simulink library "wopc_lib"  (R2024b)
settings: Solver=VariableStepAuto  StartTime=0.0  StopTime=10.0  RelTol=1e-3
undefined symbols (not defined in the file or in its folder): lambda_1, lambda_3, omega, vessel
libraries: $bdroot x13, mssSimulink x2
settings Model: Creator=lenna  LastModifiedBy=lenna

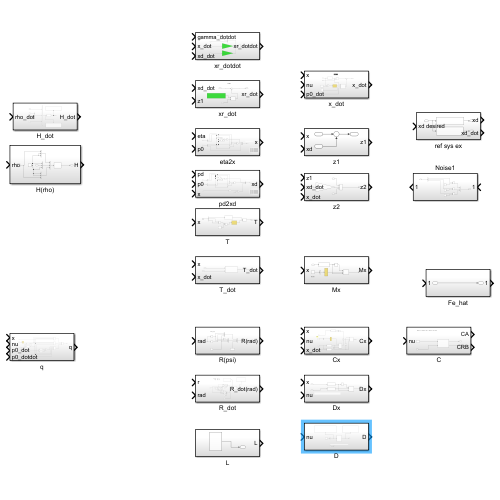
[thumbnail: Simulink's stored preview of the top-level diagram]
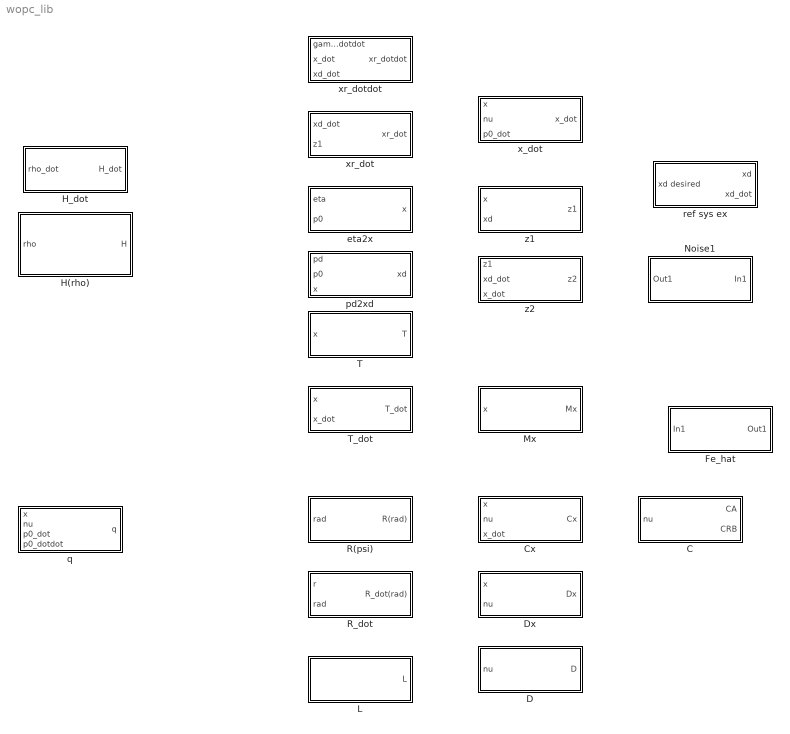
== system wopc_lib ==
  C : Subsystem
  Cx : Subsystem
  D : Subsystem
  Dx : Subsystem
  Fe_hat : Subsystem
  H(rho) : Subsystem
  H_dot : Subsystem
  L : Subsystem
  Mx : Subsystem
  Noise1 : Subsystem
  R(psi) : Subsystem
  R_dot : Subsystem
  T : Subsystem
  T_dot : Subsystem
  eta2x : Subsystem
  pd2xd : Subsystem
  q : Subsystem
  ref sys ex : Subsystem
  x_dot : Subsystem
  xr_dot : Subsystem
  xr_dotdot : Subsystem
  z1 : Subsystem
  z2 : Subsystem

== system wopc_lib/C ==
  note: Based on SIMOsv but reduced to 3DOF
  nu : Inport
  Constant : Constant  Value=vessel  OutDataTypeStr=Bus: slBus1
  Coriolis : MATLAB Function  TreatAsAtomicUnit=on
  CA : Outport
  CRB : Outport  Port=2
  wires:
  Constant/1 -> Coriolis/1(vessel)
  nu/1 -> Coriolis/2(nu)
  Coriolis/2(CRB) -> CRB/1
  Coriolis/1(CA) -> CA/1

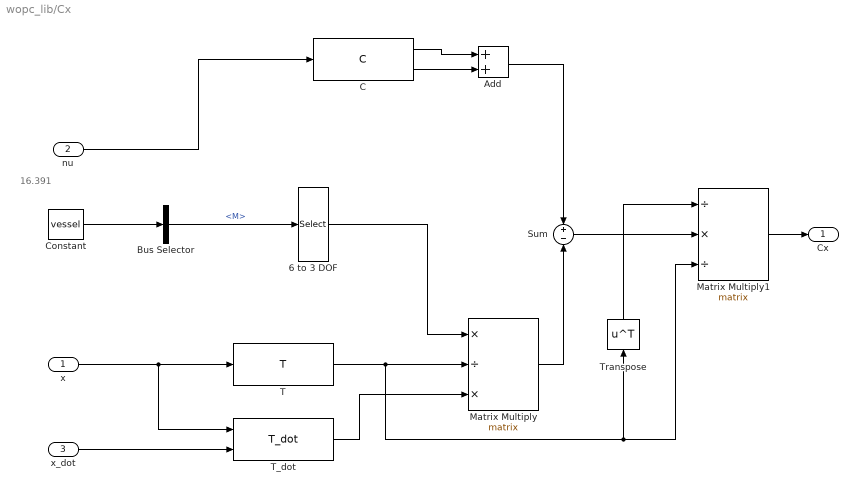
== system wopc_lib/Cx ==
  note: 16.391
  x : Inport
  nu : Inport  Port=2  PortDimensions=3
  x_dot : Inport  Port=3
  " T" : $bdroot/T  SystemSampleTime=-1  VariantActivationTime=update diagram  AllowFlexibleInterface=on  Latency=0  AutoFrameSizeCalculation=off
  6 to 3 DOF : Selector  NumberOfDimensions=2  InputPortWidth=6  IndexOptions=Index vector (dialog),Index vector (dialog)  Indices=[1 2 6],[1 2 6]  OutputSizes=1,1
  Add : Sum
  Bus Selector : BusSelector  OutputSignals=M
  C : $bdroot/C  SystemSampleTime=-1  VariantActivationTime=update diagram  AllowFlexibleInterface=on  Latency=0  AutoFrameSizeCalculation=off
  Constant : Constant  Value=vessel  OutDataTypeStr=Bus: slBus1
  Matrix Multiply : Product  Inputs=*/*  Multiplication=Matrix(*)
  Matrix Multiply1 : Product  Inputs=/*/  Multiplication=Matrix(*)
  Sum : Sum  Inputs=+-
  T_dot : $bdroot/T_dot  SystemSampleTime=-1  VariantActivationTime=update diagram  AllowFlexibleInterface=on  Latency=0  AutoFrameSizeCalculation=off
  Transpose : Math  Operator=transpose
  Cx : Outport
  wires:
  x/1 -> " T"/1, T_dot/1
  " T"/1 -> Transpose/1, Matrix Multiply1/3, Matrix Multiply/2
  6 to 3 DOF/1 -> Matrix Multiply/1
  nu/1 -> C/1
  Bus Selector/1 -> 6 to 3 DOF/1  "<M>"
  Constant/1 -> Bus Selector/1
  Matrix Multiply/1 -> Sum/2
  Matrix Multiply1/1 -> Cx/1
  Transpose/1 -> Matrix Multiply1/1
  Sum/1 -> Matrix Multiply1/2
  T_dot/1 -> Matrix Multiply/3
  x_dot/1 -> T_dot/2
  C/2 -> Add/2
  C/1 -> Add/1
  Add/1 -> Sum/1

== system wopc_lib/D ==
  note: todo: implement quadratic damping. Split d(nu) (6.116) integrals and combine with D
  nu : Inport
  Bus Selector : BusSelector  OutputSignals=D
  Constant : Constant  Value=vessel  OutDataTypeStr=Bus: slBus1
  Display : Display
  Display1 : Display
  Selector : Selector  NumberOfDimensions=2  InputPortWidth=3  IndexOptions=Index vector (dialog),Index vector (dialog)  Indices=[1 2 6],[1 2 6]  OutputSizes=1,1
  Terminator : Terminator
  D : Outport
  wires:
  Constant/1 -> Bus Selector/1
  Bus Selector/1 -> Selector/1, Display/1  "<D>"
  Selector/1 -> Display1/1, D/1
  nu/1 -> Terminator/1

== system wopc_lib/Dx ==
  note: Nonlinear D(nu) med crossflow drag og surge damping er ikke implementert.
      | Kun lineær D matrise fra osv model
  x : Inport
  nu : Inport  Port=2
  D : $bdroot/D  SystemSampleTime=-1  VariantActivationTime=update diagram  AllowFlexibleInterface=on  Latency=0  AutoFrameSizeCalculation=off
  Matrix Multiply : Product  Inputs=/*/  Multiplication=Matrix(*)
  T : $bdroot/T  SystemSampleTime=-1  VariantActivationTime=update diagram  AllowFlexibleInterface=on  Latency=0  AutoFrameSizeCalculation=off
  Transpose : Math  Operator=transpose
  Dx : Outport
  wires:
  x/1 -> T/1
  D/1 -> Matrix Multiply/2
  T/1 -> Matrix Multiply/3, Transpose/1
  Transpose/1 -> Matrix Multiply/1
  Matrix Multiply/1 -> Dx/1
  nu/1 -> D/1

== system wopc_lib/Fe_hat ==
  In1 : Inport
  Out1 : Outport
  wires:
  In1/1 -> Out1/1

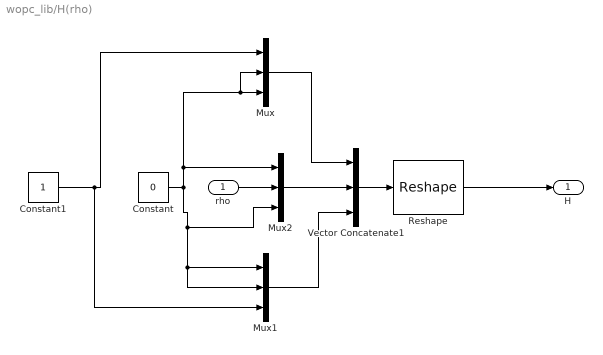
== system wopc_lib/H(rho) ==
  rho : Inport
  Constant : Constant  Value=0
  Constant1 : Constant
  Mux : Mux  Inputs=3
  Mux1 : Mux  Inputs=3
  Mux2 : Mux  Inputs=3
  Reshape : Reshape  OutputDimensionality=Customize  OutputDimensions=[3,3]
  Vector Concatenate1 : Concatenate  NumInputs=3
  H : Outport
  wires:
  Constant1/1 -> Mux1/3, Mux/1
  Constant/1 -> Mux/2, Mux/3, Mux2/1, Mux2/3, Mux1/1, Mux1/2
  Vector Concatenate1/1 -> Reshape/1
  Mux/1 -> Vector Concatenate1/1
  rho/1 -> Mux2/2
  Mux2/1 -> Vector Concatenate1/2
  Mux1/1 -> Vector Concatenate1/3
  Reshape/1 -> H/1

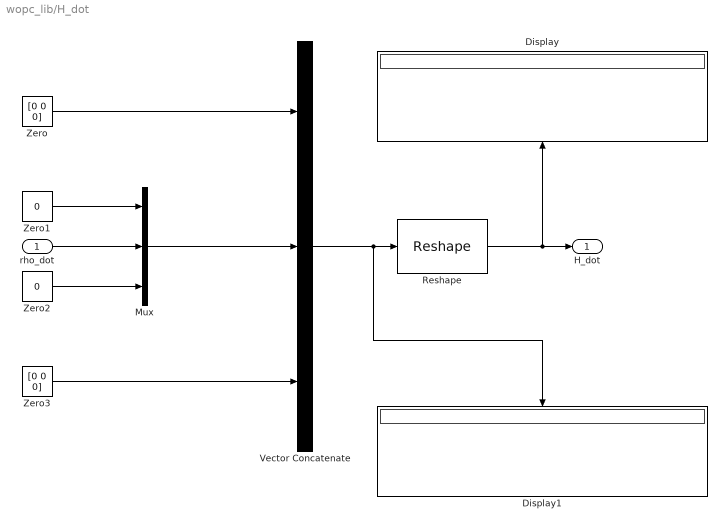
== system wopc_lib/H_dot ==
  rho_dot : Inport
  Display : Display
  Display1 : Display
  Mux : Mux  Inputs=3
  Reshape : Reshape  OutputDimensionality=Customize  OutputDimensions=[3,3]
  Vector Concatenate : Concatenate  NumInputs=3
  Zero : Constant  Value=[0 0 0]  OutDataTypeStr=Inherit: Inherit via back propagation
  Zero1 : Constant  Value=0  OutDataTypeStr=Inherit: Inherit via back propagation
  Zero2 : Constant  Value=0  OutDataTypeStr=Inherit: Inherit via back propagation
  Zero3 : Constant  Value=[0 0 0]  OutDataTypeStr=Inherit: Inherit via back propagation
  H_dot : Outport
  wires:
  Zero/1 -> Vector Concatenate/1
  Zero1/1 -> Mux/1
  rho_dot/1 -> Mux/2
  Zero2/1 -> Mux/3
  Mux/1 -> Vector Concatenate/2
  Zero3/1 -> Vector Concatenate/3
  Vector Concatenate/1 -> Display1/1, Reshape/1
  Reshape/1 -> H_dot/1, Display/1

== system wopc_lib/L ==
  L matrix : Constant  Value=[1 0;0 1;0 0]
  L : Outport
  wires:
  L matrix/1 -> L/1

== system wopc_lib/Mx ==
  note: 16.391
  x : Inport
  6 to 3 DOF : Selector  NumberOfDimensions=2  InputPortWidth=6  IndexOptions=Index vector (dialog),Index vector (dialog)  Indices=[1 2 6],[1 2 6]  OutputSizes=1,1
  Bus Selector : BusSelector  OutputSignals=M
  Constant : Constant  Value=vessel  OutDataTypeStr=Bus: slBus1
  Matrix Multiply : Product  Inputs=/*/  Multiplication=Matrix(*)
  T1 : $bdroot/T  SystemSampleTime=-1  VariantActivationTime=update diagram  AllowFlexibleInterface=on  Latency=0  AutoFrameSizeCalculation=off
  Transpose : Math  Operator=transpose
  Mx : Outport
  wires:
  6 to 3 DOF/1 -> Matrix Multiply/2  "M"
  x/1 -> T1/1
  T1/1 -> Matrix Multiply/3, Transpose/1  "T"
  Constant/1 -> Bus Selector/1
  Bus Selector/1 -> 6 to 3 DOF/1  "<M>"
  Transpose/1 -> Matrix Multiply/1  "T transp"
  Matrix Multiply/1 -> Mx/1

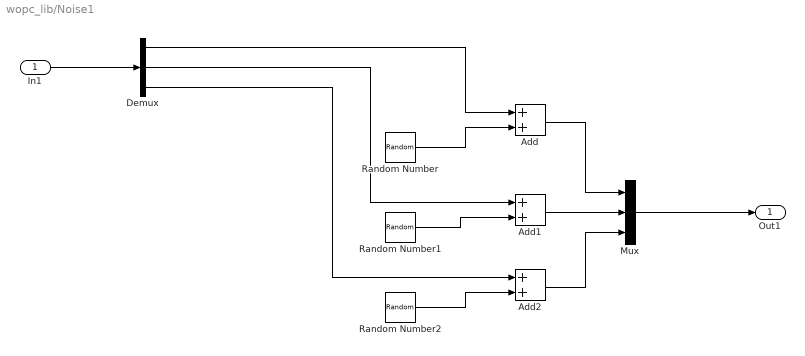
== system wopc_lib/Noise1 ==
  In1 : Inport
  Add : Sum
  Add1 : Sum
  Add2 : Sum
  Demux : Demux  Outputs=3
  Mux : Mux  Inputs=3
  Random Number : RandomNumber  Variance=0.0001^2  SampleTime=0.1
  Random Number1 : RandomNumber  Variance=0.0001^2  Seed=1  SampleTime=0.1
  Random Number2 : RandomNumber  Variance=0.0001^2  Seed=2  SampleTime=0.1
  Out1 : Outport
  wires:
  Mux/1 -> Out1/1
  Add2/1 -> Mux/3
  Add/1 -> Mux/1
  Add1/1 -> Mux/2
  Demux/3 -> Add2/1
  Demux/2 -> Add1/1
  Random Number2/1 -> Add2/2
  Random Number1/1 -> Add1/2
  Demux/1 -> Add/1
  Random Number/1 -> Add/2
  In1/1 -> Demux/1

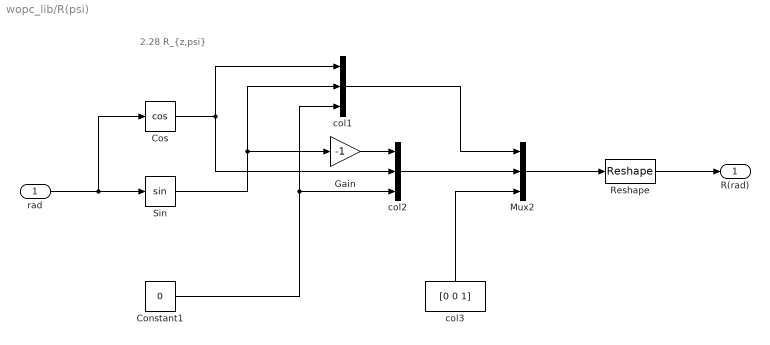
== system wopc_lib/R(psi) ==
  note: 2.28 R_{z,psi}
  rad : Inport
  Constant1 : Constant  Value=0
  Cos : Trigonometry  Operator=cos
  Gain : Gain  Gain=-1
  Mux2 : Mux  Inputs=3
  Reshape : Reshape  OutputDimensionality=Customize  OutputDimensions=[3,3]
  Sin : Trigonometry
  col1 : Mux  Inputs=3
  col2 : Mux  Inputs=3
  col3 : Constant  Value=[0 0 1]
  R(rad) : Outport
  wires:
  rad/1 -> Sin/1, Cos/1
  col3/1 -> Mux2/3
  Mux2/1 -> Reshape/1
  Reshape/1 -> R(rad)/1
  Cos/1 -> col2/2, col1/1
  Sin/1 -> col1/2, Gain/1
  Gain/1 -> col2/1
  Constant1/1 -> col1/3, col2/3
  col1/1 -> Mux2/1
  col2/1 -> Mux2/2

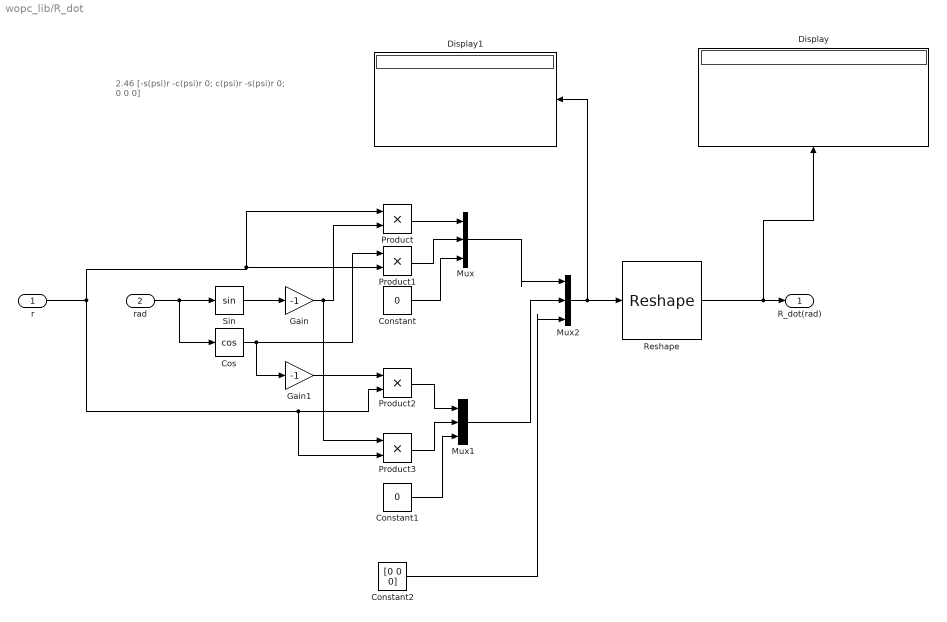
== system wopc_lib/R_dot ==
  note: 2.46 [-s(psi)r -c(psi)r 0;
      | c(psi)r -s(psi)r 0;
      | 0 0 0]
  r : Inport
  rad : Inport  Port=2
  Constant : Constant  Value=0
  Constant1 : Constant  Value=0
  Constant2 : Constant  Value=[0 0 0]
  Cos : Trigonometry  Operator=cos
  Display : Display
  Display1 : Display
  Gain : Gain  Gain=-1
  Gain1 : Gain  Gain=-1
  Mux : Mux  Inputs=3
  Mux1 : Mux  Inputs=3
  Mux2 : Mux  Inputs=3
  Product{,1..3} (4 alike) : Product
  Reshape : Reshape  OutputDimensionality=Customize  OutputDimensions=[3,3]
  Sin : Trigonometry
  R_dot(rad) : Outport
  wires:
  rad/1 -> Cos/1, Sin/1
  Sin/1 -> Gain/1
  r/1 -> Product3/2, Product2/2, Product/1, Product1/2
  Gain/1 -> Product3/1, Product/2
  Cos/1 -> Gain1/1, Product1/1
  Product/1 -> Mux/1
  Product1/1 -> Mux/2
  Constant/1 -> Mux/3
  Gain1/1 -> Product2/1
  Product2/1 -> Mux1/1
  Product3/1 -> Mux1/2
  Constant1/1 -> Mux1/3
  Mux/1 -> Mux2/1
  Mux1/1 -> Mux2/2
  Constant2/1 -> Mux2/3
  Mux2/1 -> Display1/1, Reshape/1
  Reshape/1 -> R_dot(rad)/1, Display/1

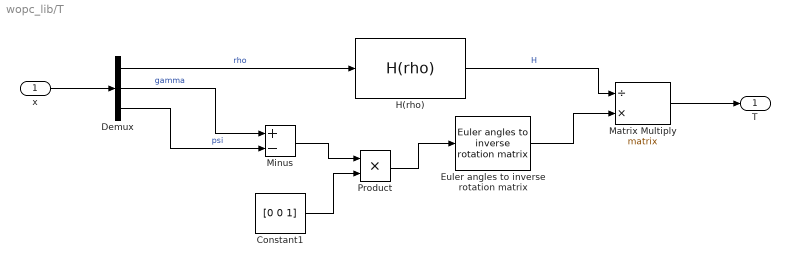
== system wopc_lib/T ==
  x : Inport
  Constant1 : Constant  Value=[0 0 1]
  Demux : Demux  Outputs=3
  Euler angles to inverse rotation matrix : mssSimulink/Modelling/Kinematics/Euler angles to inverse rotation matrix
      settings: SourceProductName=mss Toolbox
  H(rho) : $bdroot/H(rho)  SystemSampleTime=-1  VariantActivationTime=update diagram  AllowFlexibleInterface=on  Latency=0  AutoFrameSizeCalculation=off
  Matrix Multiply : Product  Inputs=/*  Multiplication=Matrix(*)
  Minus : Sum  Inputs=+-
  Product : Product
  T : Outport
  wires:
  Constant1/1 -> Product/2
  Euler angles to inverse rotation matrix/1 -> Matrix Multiply/2
  Product/1 -> Euler angles to inverse rotation matrix/1
  Demux/1 -> H(rho)/1  "rho"
  H(rho)/1 -> Matrix Multiply/1  "H"
  Demux/2 -> Minus/1  "gamma"
  Minus/1 -> Product/1
  Demux/3 -> Minus/2  "psi"
  x/1 -> Demux/1
  Matrix Multiply/1 -> T/1

== system wopc_lib/T_dot ==
  x : Inport
  x_dot : Inport  Port=2
  T_dot matrix : MATLAB Function  TreatAsAtomicUnit=on
  T_dot : Outport
  wires:
  x/1 -> T_dot matrix/1(x)  "x"
  x_dot/1 -> T_dot matrix/2(x_dot)  "x_dot"
  T_dot matrix/1(Tdot) -> T_dot/1

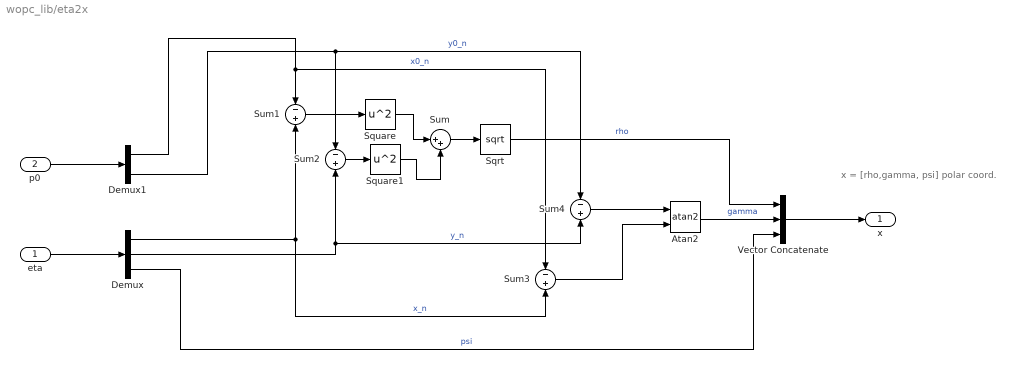
== system wopc_lib/eta2x ==
  note: x = [rho,gamma, psi] polar coord.
  eta : Inport
  p0 : Inport  Port=2
  Atan2 : Trigonometry  Operator=atan2
  Demux : Demux  Outputs=3
  Demux1 : Demux  Outputs=2
  Sqrt : Sqrt
  Square : Math  Operator=square
  Square1 : Math  Operator=square
  Sum : Sum  Inputs=|++
  Sum{1..4} (4 alike) : Sum  Inputs=-+
  Vector Concatenate : Concatenate  NumInputs=3
  x : Outport
  wires:
  Atan2/1 -> Vector Concatenate/2  "gamma"
  Sqrt/1 -> Vector Concatenate/1  "rho"
  Vector Concatenate/1 -> x/1
  eta/1 -> Demux/1
  Demux/3 -> Vector Concatenate/3  "psi"
  p0/1 -> Demux1/1
  Demux1/1 -> Sum3/1, Sum1/1  "x0_n"
  Demux/1 -> Sum3/2, Sum1/2  "x_n"
  Demux1/2 -> Sum4/1, Sum2/1  "y0_n"
  Demux/2 -> Sum4/2, Sum2/2  "y_n"
  Sum1/1 -> Square/1
  Sum2/1 -> Square1/1
  Square/1 -> Sum/1
  Square1/1 -> Sum/2
  Sum/1 -> Sqrt/1
  Sum4/1 -> Atan2/1
  Sum3/1 -> Atan2/2

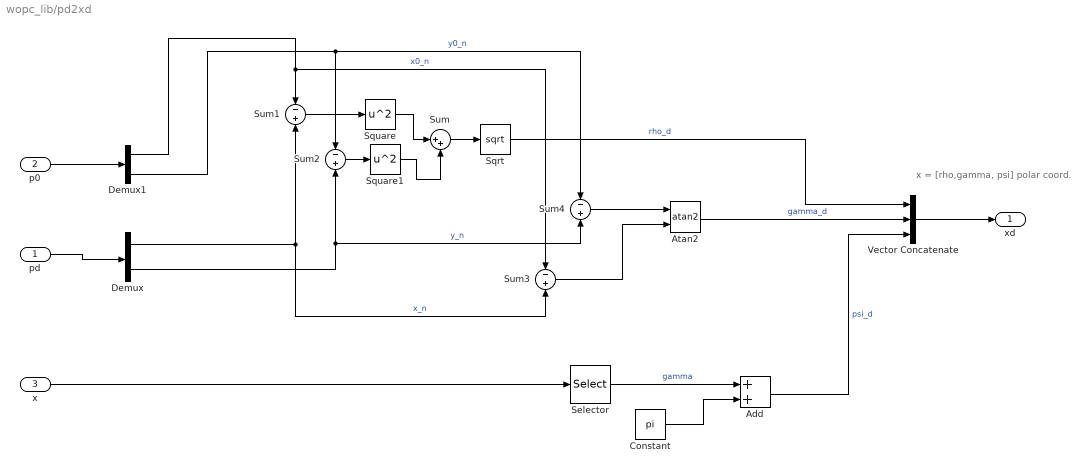
== system wopc_lib/pd2xd ==
  note: x = [rho,gamma, psi] polar coord.
  pd : Inport
  p0 : Inport  Port=2
  x : Inport  Port=3
  Add : Sum
  Atan2 : Trigonometry  Operator=atan2
  Constant : Constant  Value=pi
  Demux : Demux  Outputs=2
  Demux1 : Demux  Outputs=2
  Selector : Selector  InputPortWidth=3  IndexOptions=Index vector (dialog)  Indices=3  OutputSizes=1
  Sqrt : Sqrt
  Square : Math  Operator=square
  Square1 : Math  Operator=square
  Sum : Sum  Inputs=|++
  Sum{1..4} (4 alike) : Sum  Inputs=-+
  Vector Concatenate : Concatenate  NumInputs=3
  xd : Outport
  wires:
  Sum3/1 -> Atan2/2
  Sum4/1 -> Atan2/1
  Sum/1 -> Sqrt/1
  Square1/1 -> Sum/2
  Square/1 -> Sum/1
  Sum2/1 -> Square1/1
  Sum1/1 -> Square/1
  Demux/2 -> Sum2/2, Sum4/2  "y_n"
  Demux1/2 -> Sum2/1, Sum4/1  "y0_n"
  Demux/1 -> Sum1/2, Sum3/2  "x_n"
  Demux1/1 -> Sum1/1, Sum3/1  "x0_n"
  p0/1 -> Demux1/1
  pd/1 -> Demux/1
  Vector Concatenate/1 -> xd/1
  Sqrt/1 -> Vector Concatenate/1  "rho_d"
  Atan2/1 -> Vector Concatenate/2  "gamma_d"
  Constant/1 -> Add/2
  Add/1 -> Vector Concatenate/3  "psi_d"
  x/1 -> Selector/1
  Selector/1 -> Add/1  "gamma"

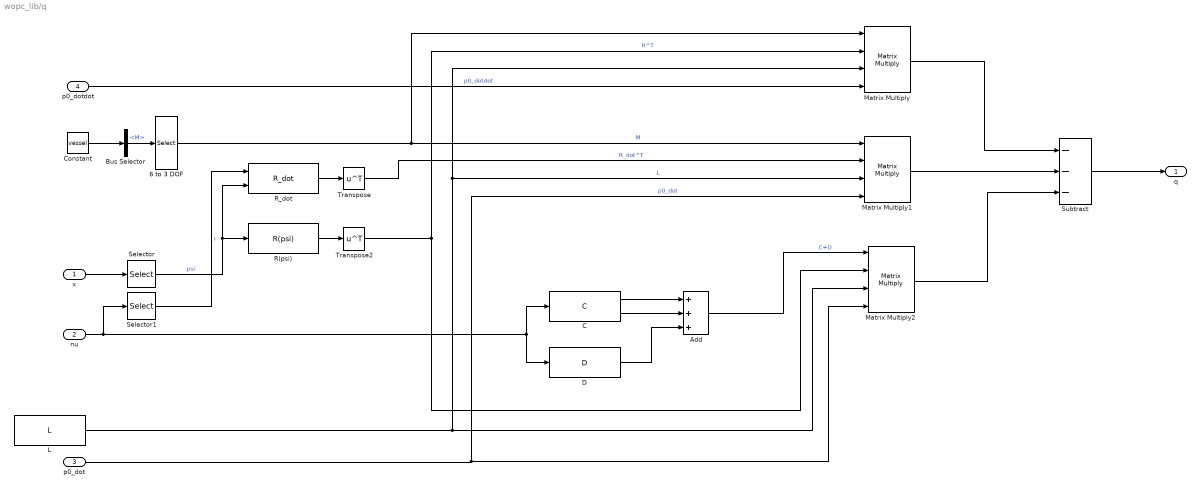
== system wopc_lib/q ==
  x : Inport
  nu : Inport  Port=2
  p0_dot : Inport  Port=3
  p0_dotdot : Inport  Port=4
  6 to 3 DOF : Selector  NumberOfDimensions=2  InputPortWidth=6  IndexOptions=Index vector (dialog),Index vector (dialog)  Indices=[1 2 6],[1 2 6]  OutputSizes=1,1
  Add : Sum  Inputs=+++
  Bus Selector : BusSelector  OutputSignals=M
  C : $bdroot/C  SystemSampleTime=-1  VariantActivationTime=update diagram  AllowFlexibleInterface=on  Latency=0  AutoFrameSizeCalculation=off
  Constant : Constant  Value=vessel  OutDataTypeStr=Bus: slBus1
  D : $bdroot/D  SystemSampleTime=-1  VariantActivationTime=update diagram  AllowFlexibleInterface=on  Latency=0  AutoFrameSizeCalculation=off
  L : $bdroot/L  SystemSampleTime=-1  VariantActivationTime=update diagram  AllowFlexibleInterface=on  Latency=0  AutoFrameSizeCalculation=off
  Matrix Multiply : Product  Inputs=4  Multiplication=Matrix(*)
  Matrix Multiply1 : Product  Inputs=4  Multiplication=Matrix(*)
  Matrix Multiply2 : Product  Inputs=4  Multiplication=Matrix(*)
  R(psi) : $bdroot/R(psi)  SystemSampleTime=-1  VariantActivationTime=update diagram  AllowFlexibleInterface=on  Latency=0  AutoFrameSizeCalculation=off
  R_dot : $bdroot/R_dot  SystemSampleTime=-1  VariantActivationTime=update diagram  AllowFlexibleInterface=on  Latency=0  AutoFrameSizeCalculation=off
  Selector : Selector  InputPortWidth=3  IndexOptions=Index vector (dialog)  Indices=[3]  OutputSizes=1
  Selector1 : Selector  InputPortWidth=3  IndexOptions=Index vector (dialog)  Indices=[3]  OutputSizes=1
  Subtract : Sum  Inputs=---
  Transpose : Math  Operator=transpose
  Transpose2 : Math  Operator=transpose
  q : Outport
  wires:
  Bus Selector/1 -> 6 to 3 DOF/1  "<M>"
  Constant/1 -> Bus Selector/1
  6 to 3 DOF/1 -> Matrix Multiply1/1, Matrix Multiply/1  "M"
  p0_dotdot/1 -> Matrix Multiply/4  "p0_dotdot"
  R(psi)/1 -> Transpose2/1
  Selector/1 -> R(psi)/1, R_dot/2  "psi"
  Matrix Multiply/1 -> Subtract/1
  R_dot/1 -> Transpose/1
  p0_dot/1 -> Matrix Multiply1/4, Matrix Multiply2/4  "p0_dot"
  Transpose/1 -> Matrix Multiply1/2  "R_dot^T"
  L/1 -> Matrix Multiply2/3, Matrix Multiply1/3, Matrix Multiply/3  "L"
  x/1 -> Selector/1
  Transpose2/1 -> Matrix Multiply2/2, Matrix Multiply/2  "R^T"
  Matrix Multiply1/1 -> Subtract/2
  D/1 -> Add/3
  C/1 -> Add/1
  C/2 -> Add/2
  nu/1 -> Selector1/1, C/1, D/1
  Selector1/1 -> R_dot/1  "r"
  Add/1 -> Matrix Multiply2/1  "C+D"
  Matrix Multiply2/1 -> Subtract/3
  Subtract/1 -> q/1

== system wopc_lib/ref sys ex ==
  xd desired : Inport
  Transfer Fcn : TransferFcn  Denominator=[1 2*omega omega^2]
  Transfer Fcn1 : TransferFcn  Numerator=[1 0]  Denominator=[1 2*omega omega^2]
  xd : Outport
  xd_dot : Outport  Port=2
  wires:
  xd desired/1 -> Transfer Fcn/1, Transfer Fcn1/1  "xd"
  Transfer Fcn/1 -> xd/1  "xd"
  Transfer Fcn1/1 -> xd_dot/1  "xd_dot"

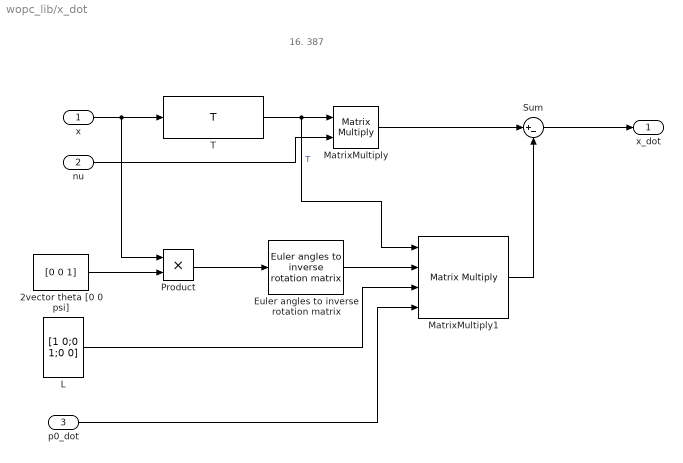
== system wopc_lib/x_dot ==
  note: 16. 387
  x : Inport
  nu : Inport  Port=2
  p0_dot : Inport  Port=3
  2vector theta [0 0 psi] : Constant  Value=[0 0 1]
  Euler angles to inverse rotation matrix : mssSimulink/Modelling/Kinematics/Euler angles to inverse rotation matrix
      settings: SourceProductName=mss Toolbox
  L : Constant  Value=[1 0;0 1;0 0]
  MatrixMultiply : Product  Multiplication=Matrix(*)
  MatrixMultiply1 : Product  Inputs=4  Multiplication=Matrix(*)
  Product : Product
  Sum : Sum  Inputs=|+-
  T : $bdroot/T  SystemSampleTime=-1  VariantActivationTime=update diagram  AllowFlexibleInterface=on  Latency=0  AutoFrameSizeCalculation=off
  x_dot : Outport
  wires:
  x/1 -> Product/1, T/1
  T/1 -> MatrixMultiply1/1, MatrixMultiply/1  "T"
  nu/1 -> MatrixMultiply/2
  MatrixMultiply/1 -> Sum/1
  Product/1 -> Euler angles to inverse rotation matrix/1
  2vector theta [0 0 psi]/1 -> Product/2
  Euler angles to inverse rotation matrix/1 -> MatrixMultiply1/2
  L/1 -> MatrixMultiply1/3
  p0_dot/1 -> MatrixMultiply1/4
  MatrixMultiply1/1 -> Sum/2
  Sum/1 -> x_dot/1

== system wopc_lib/xr_dot ==
  note: 16.397
  xd_dot : Inport
  z1 : Inport  Port=2  PortDimensions=3
  Constant : Constant  Value=[lambda_1 0 0;0 0 0;0 0 lambda_3]
  Matrix Multiply : Product  Multiplication=Matrix(*)
  Sum : Sum  Inputs=|+-
  xr_dot : Outport
  wires:
  Constant/1 -> Matrix Multiply/1
  z1/1 -> Matrix Multiply/2
  Matrix Multiply/1 -> Sum/2
  xd_dot/1 -> Sum/1
  Sum/1 -> xr_dot/1

== system wopc_lib/xr_dotdot ==
  note: derivative of 16.397
  gamma_dotdot : Inport
  x_dot : Inport  Port=2
  xd_dot : Inport  Port=3
  Constant : Constant  Value=0
  Lambda : Gain  Gain=diag([lambda_1, 0, lambda_3])  Multiplication=Matrix(K*u)
  Lambda1 : Gain  Gain=diag([lambda_1, 0, lambda_3])  Multiplication=Matrix(K*u)
  Mux : Mux  Inputs=3
  Subtract : Sum  Inputs=+-+
  xr_dotdot : Outport
  wires:
  Subtract/1 -> xr_dotdot/1
  x_dot/1 -> Lambda/1
  xd_dot/1 -> Lambda1/1
  Lambda/1 -> Subtract/2
  Lambda1/1 -> Subtract/3
  gamma_dotdot/1 -> Mux/3  "psi_d_dotdot = gamma_dotdot"
  Constant/1 -> Mux/1, Mux/2
  Mux/1 -> Subtract/1

== system wopc_lib/z1 ==
  x : Inport
  xd : Inport  Port=2
  Sum : Sum  Inputs=|+-
  z1 : Outport
  wires:
  x/1 -> Sum/1
  xd/1 -> Sum/2
  Sum/1 -> z1/1

== system wopc_lib/z2 ==
  z1 : Inport
  xd_dot : Inport  Port=2
  x_dot : Inport  Port=3
  Add : Sum  Inputs=++-
  Lambda : Gain  Gain=diag([lambda_1, 0, lambda_3])  Multiplication=Matrix(K*u)
  z2 : Outport
  wires:
  z1/1 -> Lambda/1
  Lambda/1 -> Add/2
  x_dot/1 -> Add/1
  xd_dot/1 -> Add/3
  Add/1 -> z2/1

== matlab function wopc_lib/C/Coriolis ==
  data: CA output; vessel input; CRB output; nu input size=3
function [CA, CRB]  = fcn(vessel,nu)

% CRB is only dependant on angular velocities nu2
nu2 = [0 0 nu(3)]';

% Coriolis matrices
[~,CRB6DOF] = rbody(vessel.m,vessel.R44,vessel.R55,vessel.R66,nu2,vessel.r_bg'); 

% Controller uses only 3DOF
CRB = CRB6DOF([1 2 6], [1 2 6]);

MA = vessel.MA([1 2 6], [1 2 6]);
CA  = m2c(MA, nu);

== matlab function wopc_lib/T_dot/T_dot matrix ==
  data: x input; Tdot output; x_dot input
function Tdot = fcn(x,x_dot)
% T_dot matrix derived for x = (rho,gamma,psi)
% see p619

a = x(3) - x(2);
rho = x(1);

%dT/drho
dTdr21 = sin(a)/rho^2;
dTdr22 = cos(a)/rho^2;

dTdrho = [    0,          0,            0;
            dTdr21,     dTdr22,         0;
              0,          0,            0];

% dT/dgamma
dTdg11 = -sin(a);
dTdg12 = cos(a);
dTdg21 = -cos(a)/rho;
dTdg22 = -sin(a)/rho;

dTdgamma = [
    dTdg11, dTdg12, 0;
    dTdg21, dTdg22, 0;
         0,      0, 0];

%dT/dpsi
dTdp11 = sin(a);
dTdp12 = -cos(a);
dTdp21 = cos(a)/rho;
dTdp22 = sin(a)/rho;

dTdpsi = [
    dTdp11, dTdp12, 0;
    dTdp21, dTdp22, 0;
         0,      0, 0];

Tdot = dTdrho * x_dot(1) + dTdgamma * x_dot(2) + dTdpsi * x_dot(3);
